simulink model "LQG"  (R2022b)
settings: Solver=VariableStepAuto  StartTime=0.0  StopTime=10  RelTol=1e-3
values from neighbouring files (symbols this model uses):
  A_an = P_attuato.A    [Progetto_CSI.m]
  B_an = P_attuato.B    [Progetto_CSI.m]
  C_an = P_attuato.C    [Progetto_CSI.m]
  cond_iniz = [teta0(1);teta0(2);dteta0(1);dteta0(2)]    [Progetto_CSI.m]
  Kf = lqe(A_an,Bnoise,C_an,W,V)    [Progetto_CSI.m]
  Km1 = ureal('Km1',1.08,'Percentage',10)    [Progetto_CSI.m]
  Km2 = ureal('Km2',0.335,'Percentage',10)    [Progetto_CSI.m]
  Kr = lqr(Aaum,Baum,Q,R)    [Progetto_CSI.m]
  stdv_wd = 0.03    [Progetto_CSI.m]
  stdv_wn = 0.03    [Progetto_CSI.m]
  Tm1 = ureal('Tm1',0.005,'Percentage',20)    [Progetto_CSI.m]
  Tm2 = ureal('Tm2',0.002,'Percentage',20)    [Progetto_CSI.m]
settings Model: Creator=paoga  LastModifiedBy=paoga

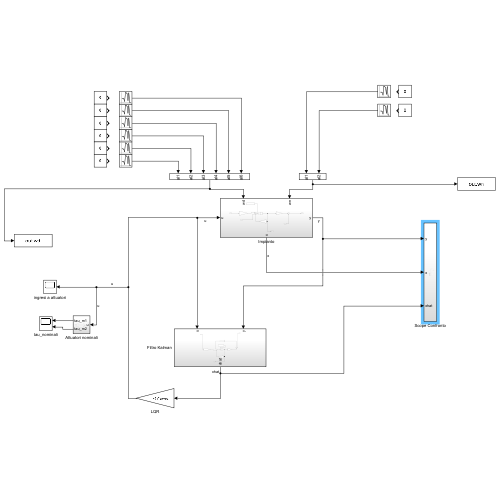
[thumbnail: Simulink's stored preview of the top-level diagram]
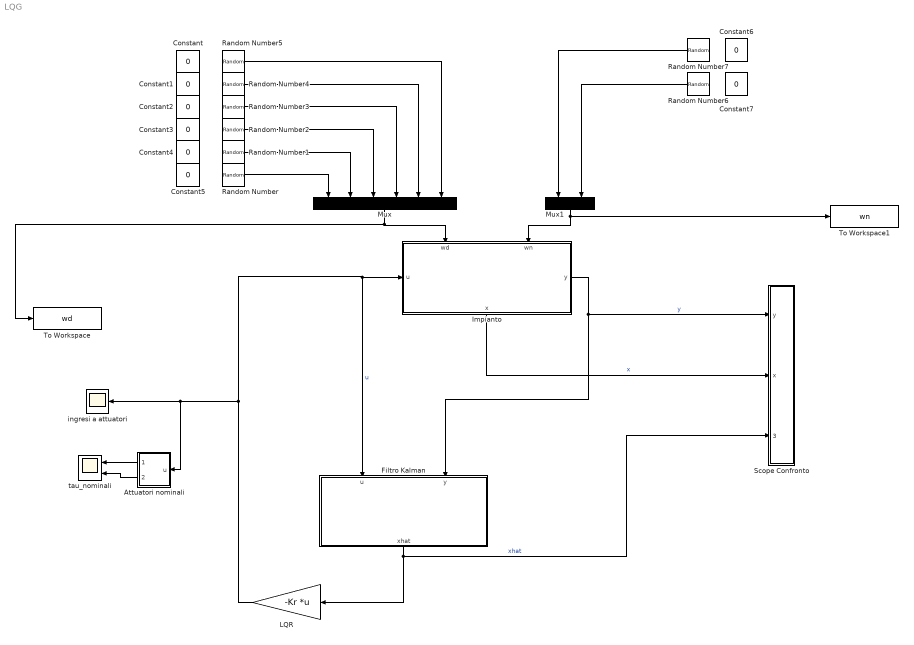
== system LQG ==
  Attuatori nominali : Subsystem
  Constant{,1..7} (8 alike) : Constant  Value=0
  Filtro Kalman : Subsystem
  Impianto : Subsystem
      settings: PortSchema="{\"entries\":[{\"content\":{\"sides\":[{\"content\":{\"connectorIds\":[\"In1\"]},\"type\":\"ConnectorPlacement.EquallySpacedRectSide\",\"uuid\":\"1f338e48-7831-4bd3-85b4-3ffb6ec30be0\"},{\"content\":{\"connectorIds\":[\"Out1\"],\"side\":\"RIGHT\"},\"type\":\"ConnectorPlacement.EquallySpacedRectSide\",\"uuid\":\"72b62bfc-b5ba-4fca-990c-fb8ade2baa52\"},{\"content\":{\"connectorIds\":[\"In2\",\"In3\"],\"side\":\"TOP\"},\"type\":\"ConnectorPlacement.EquallySpacedRectSide\",\"uuid\":\"1923cf88-f089-4e4d-b540-4a25050c7ba1\"},{\"content\":{\"connectorIds\":[\"Out2\"],\"side\":\"BOTTOM\"},\"type\":\"ConnectorPlacement.EquallySpacedRectSide\",\"uuid\":\"27a80785-b208-442b-bd38-b71cea9955a7\"}]},\"type\":\"ConnectorPlacement.EquallySpacedConnector\",\"uuid\":\"4af3c447-5e92-4354-9d25-9c8910426d40\"}],\"packageUris\":[\"http://schema.mathworks.com/mf0/Connector/R2020b\"],\"version\":\"1.0\"}"
  LQR : Gain  Gain=-Kr  Multiplication=Matrix(K*u) (u vector)
  Mux : Mux  Inputs=6
      settings: DisplayOption=signals
  Mux1 : Mux  Inputs=2
      settings: DisplayOption=signals
  Random Number{,1..5} (6 alike) : RandomNumber  Variance=stdv_wd^2  SampleTime=0.01
  Random Number6 : RandomNumber  Variance=stdv_wn^2  SampleTime=0.01
  Random Number7 : RandomNumber  Variance=stdv_wn^2  SampleTime=0.01
  Scope Confronto : Subsystem
  To Workspace : ToWorkspace  VariableName=wd  SampleTime=-1
  To Workspace1 : ToWorkspace  VariableName=wn  SampleTime=-1
  ingresi a attuatori : Scope
  tau_nominali : Scope  NumInputPorts=2
  wires:
  Filtro Kalman/1(xhat) -> Scope Confronto/3(xhat), LQR/1  "xhat"
  LQR/1 -> Impianto/1(u), Filtro Kalman/1(u), Attuatori nominali/1(u), ingresi a attuatori/1  "u"
  Impianto/1(y) -> Filtro Kalman/2(y), Scope Confronto/1(y)  "y"
  Mux/1 -> To Workspace/1, Impianto/2(wd)
  Mux1/1 -> Impianto/3(wn), To Workspace1/1
  Attuatori nominali/1(tau_m1) -> tau_nominali/1
  Attuatori nominali/2(tau_m2) -> tau_nominali/2
  Impianto/2(x) -> Scope Confronto/2(x)  "x"
  Random Number/1 -> Mux/1
  Random Number1/1 -> Mux/2
  Random Number2/1 -> Mux/3
  Random Number3/1 -> Mux/4
  Random Number4/1 -> Mux/5
  Random Number5/1 -> Mux/6
  Random Number6/1 -> Mux1/2
  Random Number7/1 -> Mux1/1

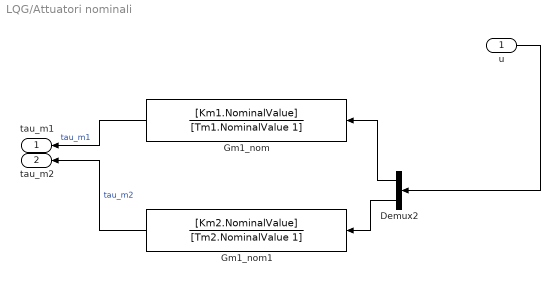
== system LQG/Attuatori nominali ==
  u : Inport
  Demux2 : Demux  Outputs=2
  Gm1_nom : TransferFcn  Numerator=[Km1.NominalValue]  Denominator=[Tm1.NominalValue 1]
  Gm1_nom1 : TransferFcn  Numerator=[Km2.NominalValue]  Denominator=[Tm2.NominalValue 1]
  tau_m1 : Outport
  tau_m2 : Outport  Port=2
  wires:
  u/1 -> Demux2/1
  Demux2/1 -> Gm1_nom/1
  Demux2/2 -> Gm1_nom1/1
  Gm1_nom/1 -> tau_m1/1  "tau_m1"
  Gm1_nom1/1 -> tau_m2/1  "tau_m2"

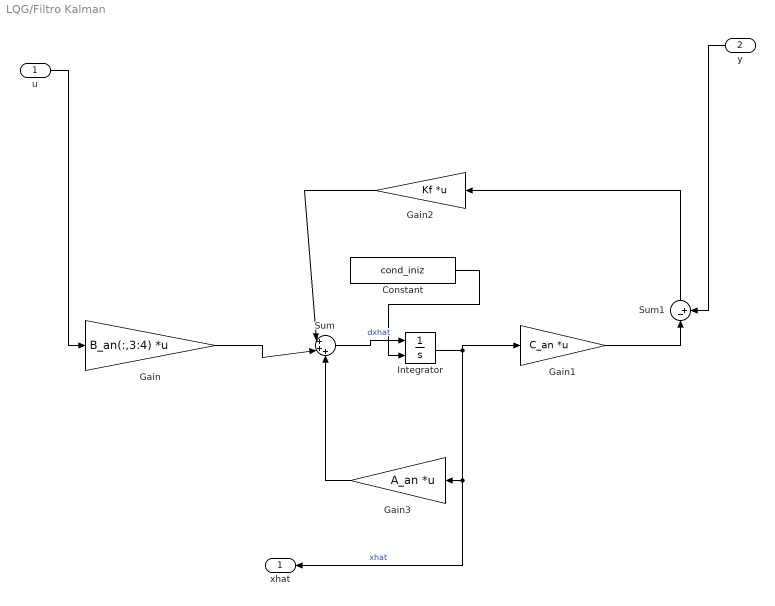
== system LQG/Filtro Kalman ==
  u : Inport
  y : Inport  Port=2
  Constant : Constant  Value=cond_iniz
  Gain : Gain  Gain=B_an(:,3:4)  Multiplication=Matrix(K*u) (u vector)
  Gain1 : Gain  Gain=C_an  Multiplication=Matrix(K*u) (u vector)
  Gain2 : Gain  Gain=Kf  Multiplication=Matrix(K*u) (u vector)
  Gain3 : Gain  Gain=A_an  Multiplication=Matrix(K*u) (u vector)
  Integrator : Integrator  InitialConditionSource=external
  Sum : Sum  Inputs=|+++
  Sum1 : Sum  Inputs=|-+
  xhat : Outport
  wires:
  Sum/1 -> Integrator/1  "dxhat"
  Gain1/1 -> Sum1/1
  Gain3/1 -> Sum/3
  Gain2/1 -> Sum/1
  Integrator/1 -> Gain1/1, xhat/1, Gain3/1  "xhat"
  Gain/1 -> Sum/2
  Sum1/1 -> Gain2/1
  u/1 -> Gain/1
  y/1 -> Sum1/2
  Constant/1 -> Integrator/2

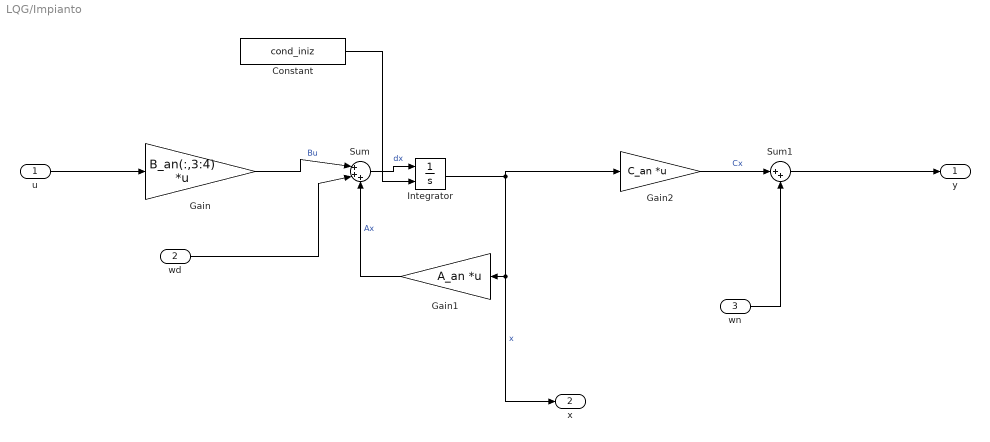
== system LQG/Impianto ==
  u : Inport
  wd : Inport  Port=2
  wn : Inport  Port=3
  Constant : Constant  Value=cond_iniz
  Gain : Gain  Gain=B_an(:,3:4)  Multiplication=Matrix(K*u) (u vector)
  Gain1 : Gain  Gain=A_an  Multiplication=Matrix(K*u) (u vector)
  Gain2 : Gain  Gain=C_an  Multiplication=Matrix(K*u) (u vector)
  Integrator : Integrator  InitialConditionSource=external  InitialCondition=[0.5;0.5;0;0;0;0]
  Sum : Sum  Inputs=|+++
  Sum1 : Sum  Inputs=|++
  y : Outport
  x : Outport  Port=2
  wires:
  u/1 -> Gain/1
  Gain/1 -> Sum/1  "Bu"
  wd/1 -> Sum/2
  Sum/1 -> Integrator/1  "dx"
  Integrator/1 -> Gain2/1, x/1, Gain1/1  "x"
  Gain1/1 -> Sum/3  "Ax"
  Gain2/1 -> Sum1/1  "Cx"
  wn/1 -> Sum1/2
  Sum1/1 -> y/1
  Constant/1 -> Integrator/2

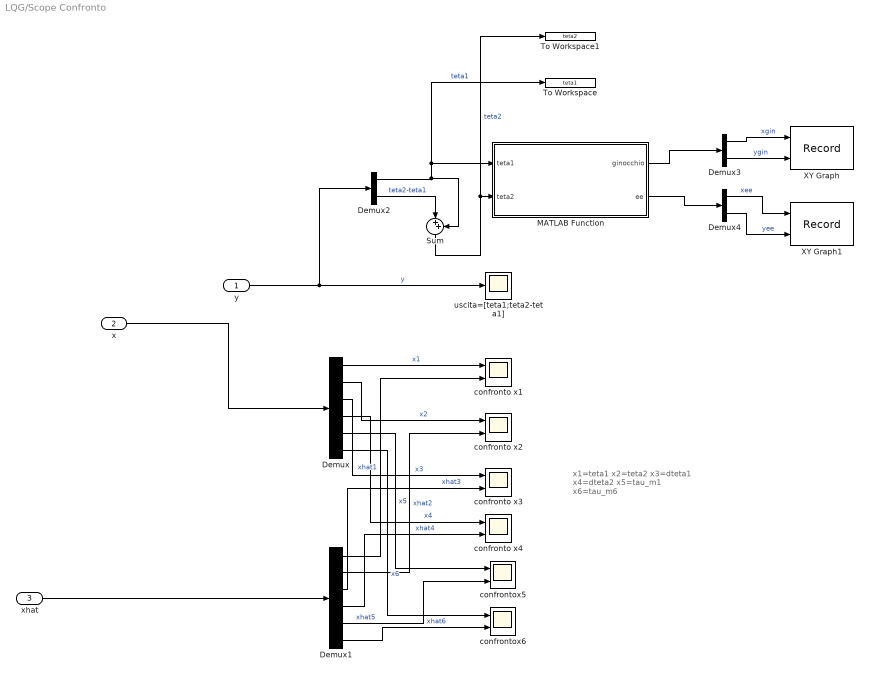
== system LQG/Scope Confronto ==
  note: x1=teta1
      | x2=teta2
      | x3=dteta1
      | x4=dteta2
      | x5=tau_m1
      | x6=tau_m6
  y : Inport
  x : Inport  Port=2
  xhat : Inport  Port=3
  Demux : Demux  Outputs=6
  Demux1 : Demux  Outputs=6
  Demux2 : Demux  Outputs=2
  Demux3 : Demux  Outputs=2
  Demux4 : Demux  Outputs=2
  MATLAB Function : MATLAB Function  TreatAsAtomicUnit=on
  Sum : Sum  Inputs=|++
  To Workspace : ToWorkspace  VariableName=teta1  SaveFormat=Timeseries  SampleTime=0.001
  To Workspace1 : ToWorkspace  VariableName=teta2  SaveFormat=Timeseries  SampleTime=0.001
  XY Graph : Record  FileSettingsInternal="{\"entries\":[{\"content\":{\"excelSettings\":{\"content\":{},\"type\":\"Streamout.ExcelSettings\"}},\"type\":\"Streamout.FileSettingStorage\",\"uuid\":\"5915aa3a-dbbf-4d6b-9ae6-d93c60de66de\"}],\"packageUris\":[\"http://schema.mathworks.com/mf0/streamout_blocks/R2020a\"],\"version\":\"1.0\"}"  Layout=[1 1]  SignalsInternal="{\"entries\":[{\"content\":{\"signals\":[{\"content\":{\"blockPath\":[\"LQG/Scope Confronto/XY Graph\"],\"channel\":[],\"dimensions\":[1,1],\"domain\":\"LQG/Scope Confronto/XY Graph\",\"lineColor\":\"#edb120\",\"plots\":[1],\"port\":1,\"sid\":[\"\"],\"signalID\":27,\"signalName\":\"xgin\"},\"type\":\"RecordBlkView.Signal\",\"uuid\":\"51e2fcfa-b634-44d6-b8f4-0fb802e549cd\"},{\"content\":{\"blockPath\":[\"LQG/Scope Confronto/XY Graph\"],\"channel\":[],\"dimensions\":[1,1],\"domain\":\"LQG/Scope Confronto/XY Graph\",\"lineColor\":\"#139fff\",\"plots\":[1],\"port\":2,\"sid\":[\"\"],\"signalID\":31,\"signalName\":\"ygin\"},\"type\":\"RecordBlkView.Signal\",\"uuid\":\"ec1641ea-dcb0-41b4-81a5-6fb14d69c143\"}]},\"type\":\"RecordBlkView.InputSignals\",\"uuid\":\"84637c77-13ae-4712-99ea-852f35c05741\"}],\"packageUris\":[\"http://schema.mathworks.com/mf0/streamout_blocks/R2020a\"],\"version\":\"1.0\"}"  VisualizationBindings="{\"sparklinesplugin\":{\"info\":[{\"bindingParametersList\":[],\"subplotID\":1}]}}"  CompatibilityTag=XY
  XY Graph1 : Record  FileSettingsInternal="{\"entries\":[{\"content\":{\"excelSettings\":{\"content\":{},\"type\":\"Streamout.ExcelSettings\"}},\"type\":\"Streamout.FileSettingStorage\",\"uuid\":\"a0a548bb-86c5-496d-8a7c-88a2b02bf6a4\"}],\"packageUris\":[\"http://schema.mathworks.com/mf0/streamout_blocks/R2020a\"],\"version\":\"1.0\"}"  Layout=[1 1]  SignalsInternal="{\"entries\":[{\"content\":{\"signals\":[{\"content\":{\"blockPath\":[\"LQG/Scope Confronto/XY Graph1\"],\"channel\":[],\"dimensions\":[1,1],\"domain\":\"LQG/Scope Confronto/XY Graph1\",\"lineColor\":\"#77ac30\",\"plots\":[1],\"port\":1,\"sid\":[\"\"],\"signalID\":35,\"signalName\":\"xee\"},\"type\":\"RecordBlkView.Signal\",\"uuid\":\"0cd7c456-dbdc-41bd-bb39-d03bd9d6deed\"},{\"content\":{\"blockPath\":[\"LQG/Scope Confronto/XY Graph1\"],\"channel\":[],\"dimensions\":[1,1],\"domain\":\"LQG/Scope Confronto/XY Graph1\",\"lineColor\":\"#64d413\",\"plots\":[1],\"port\":2,\"sid\":[\"\"],\"signalID\":39,\"signalName\":\"yee\"},\"type\":\"RecordBlkView.Signal\",\"uuid\":\"6344294f-806f-4ce9-978c-8c249122de7f\"}]},\"type\":\"RecordBlkView.InputSignals\",\"uuid\":\"762e2d5b-f691-4aeb-8ea9-c7418d32d29e\"}],\"packageUris\":[\"http://schema.mathworks.com/mf0/streamout_blocks/R2020a\"],\"version\":\"1.0\"}"  VisualizationBindings="{\"sparklinesplugin\":{\"info\":[{\"bindingParametersList\":[],\"subplotID\":1}]}}"  CompatibilityTag=XY
  confronto x{1..4} (4 alike) : Scope  NumInputPorts=2
  confrontox5 : Scope  NumInputPorts=2
  confrontox6 : Scope  NumInputPorts=2
  uscita=[teta1;teta2-teta1] : Scope
  wires:
  Demux1/5 -> confrontox5/2  "xhat5"
  Demux/1 -> confronto x1/1  "x1"
  Demux1/6 -> confrontox6/2  "xhat6"
  Demux/6 -> confrontox6/1  "x6"
  Demux1/2 -> confronto x2/2  "xhat2"
  Demux1/1 -> confronto x1/2  "xhat1"
  Demux1/4 -> confronto x4/2  "xhat4"
  Demux/4 -> confronto x4/1  "x4"
  Demux1/3 -> confronto x3/2  "xhat3"
  Demux/5 -> confrontox5/1  "x5"
  Demux/2 -> confronto x2/1  "x2"
  Demux/3 -> confronto x3/1  "x3"
  x/1 -> Demux/1
  xhat/1 -> Demux1/1
  Demux4/2 -> XY Graph1/2  "yee"
  MATLAB Function/2(ee) -> Demux4/1
  MATLAB Function/1(ginocchio) -> Demux3/1
  Demux2/2 -> Sum/1  "teta2-teta1"
  Demux3/1 -> XY Graph/1  "xgin"
  y/1 -> uscita=[teta1;teta2-teta1]/1, Demux2/1  "y"
  Demux3/2 -> XY Graph/2  "ygin"
  Demux4/1 -> XY Graph1/1  "xee"
  Sum/1 -> MATLAB Function/2(teta2), To Workspace1/1  "teta2"
  Demux2/1 -> To Workspace/1, MATLAB Function/1(teta1), Sum/2  "teta1"

== matlab function LQG/Scope Confronto/MATLAB Function ==
  data: teta1 input; ginocchio output; teta2 input; ee output
function [ginocchio,ee] = fcn(teta1,teta2)
l1=0.5;l2=0.4;
ginocchio=[l1*sin(teta1);
           l1*cos(teta1)];
ee=ginocchio+[l2*sin(teta2);
           l2*cos(teta2)];
end
